simulink model "motor_start"  (R2021b)
settings: Solver=VariableStepAuto  StartTime=0.0  StopTime=10.0  RelTol=1e-3
settings Model: Creator=cirie  LastModifiedBy=cirie

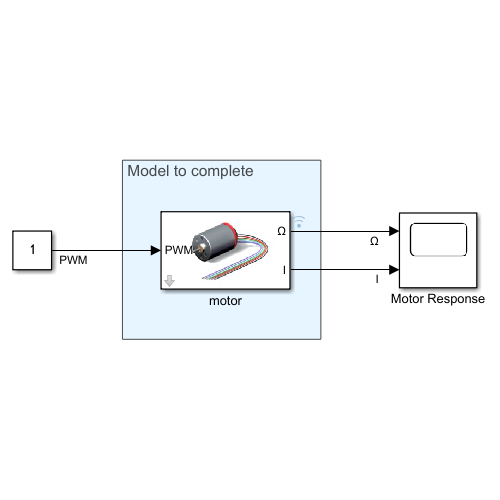
[thumbnail: Simulink's stored preview of the top-level diagram]
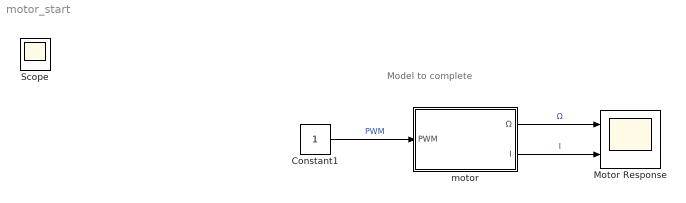
== system motor_start ==
  note: Model to complete
  Constant1 : Constant
  Motor Response : Scope  NumInputPorts=2
  motor : Subsystem  mask(DC Motor){J=1e-4, km=0.1, R=1, Vmax=7.2}
      mask prompts: J "Inertia, J [kgm^2]"; km "Motor constant, km [V*s/rad]"; R "Resistance, R [Ohm]"; Vmax "Maximum Voltage, Vmax [V]"
      mask help:
      | Circuit Dynamics:   PWM*Vmax == I*R + km*Ω
      | Rotor Dynamics:     J*dΩ/dt == km*I
      mask Display: image('$imagefile'); % Use "Edit Image" on toolstrip to change.
  Scope : Scope
  wires:
  Constant1/1 -> motor/1(PWM)  "PWM"
  motor/1(Ω) -> Motor Response/1  "Ω"
  motor/2(I) -> Motor Response/2  "I"

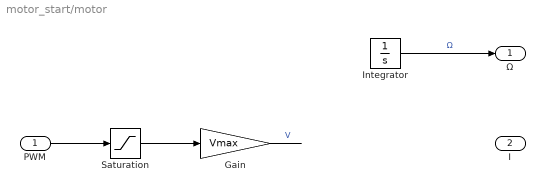
== system motor_start/motor ==
  PWM : Inport
  Gain : Gain  Gain=Vmax
  Integrator : Integrator
  Saturation : Saturate  UpperLimit=1  LowerLimit=-1
  Ω : Outport
  I : Outport  Port=2
  wires:
  ? -> Integrator/1  "dΩ/dt"
  Integrator/1 -> Ω/1  "Ω"
  ? -> I/1  "I"
  PWM/1 -> Saturation/1
  Gain/1 -> ?  "V"
  Saturation/1 -> Gain/1
